simulink model "ejercicio51listo"  (R2017a)
settings: Solver=FixedStepAuto  StartTime=0.0  StopTime=3  FixedStep=1e-6  RelTol=1e-3
undefined symbols (not defined in the file): filtrovco
libraries: dsparch4 x2, commsynccomp2 x1
settings Model: Creator=Nahuel  LastModifiedBy=gusta

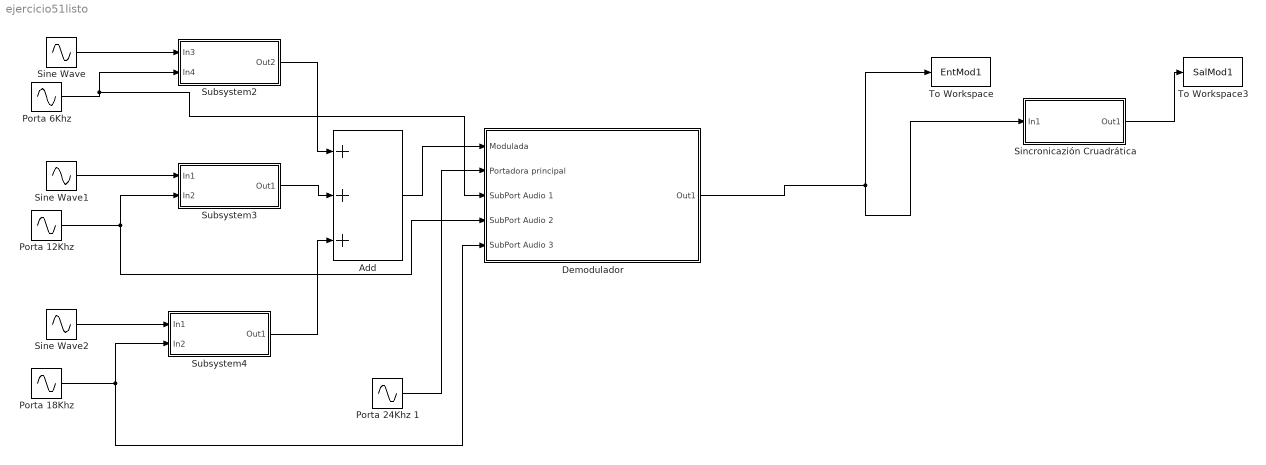
== system ejercicio51listo ==
  Add : Sum  Inputs=+++
  Demodulador : Subsystem
  "Porta 12Khz " : Sin  Frequency=2*pi*12000
  "Porta 18Khz " : Sin  Frequency=2*pi*18000
  Porta 24Khz 1 : Sin  Frequency=2*pi*24000
  "Porta 6Khz " : Sin  Frequency=2*pi*6000
  Sincronicazión Cruadrática : Subsystem
  Sine Wave : Sin  Frequency=100*pi*2  Phase=pi/2
  Sine Wave1 : Sin  Frequency=500*pi*2  Phase=pi/2
  Sine Wave2 : Sin  Frequency=250*pi*2  Phase=pi/2
  Subsystem2 : Subsystem
  Subsystem3 : Subsystem
  Subsystem4 : Subsystem
  To Workspace : ToWorkspace  VariableName=EntMod1  SampleTime=-1
  To Workspace3 : ToWorkspace  VariableName=SalMod1  SampleTime=-1
  wires:
  Demodulador/1(Out1) -> Sincronicazión Cruadrática/1(In1), To Workspace/1
  Sincronicazión Cruadrática/1(Out1) -> To Workspace3/1
  "Porta 6Khz "/1 -> Demodulador/3(SubPort Audio 1), Subsystem2/2(In4)
  Sine Wave/1 -> Subsystem2/1(In3)
  Subsystem2/1(Out2) -> Add/1
  Subsystem3/1(Out1) -> Add/2
  "Porta 12Khz "/1 -> Subsystem3/2(In2), Demodulador/4(SubPort Audio 2)
  Sine Wave1/1 -> Subsystem3/1(In1)
  Subsystem4/1(Out1) -> Add/3
  Sine Wave2/1 -> Subsystem4/1(In1)
  "Porta 18Khz "/1 -> Demodulador/5(SubPort Audio 3), Subsystem4/2(In2)
  Porta 24Khz 1/1 -> Demodulador/2(Portadora principal)
  Add/1 -> Demodulador/1(Modulada)

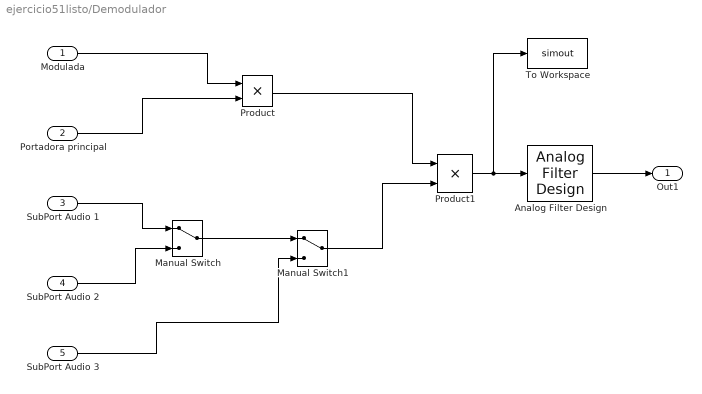
== system ejercicio51listo/Demodulador ==
  Modulada : Inport
  Portadora principal : Inport  Port=2
  SubPort Audio 1 : Inport  Port=3
  SubPort Audio 2 : Inport  Port=4
  SubPort Audio 3 : Inport  Port=5
  Analog Filter Design : dsparch4/Analog Filter Design  method=Butterworth  filttype=Lowpass  N=12  Wlo=2*pi*5000  Whi=80  Rp=2  Rs=40
  Manual Switch : ManualSwitch
  Manual Switch1 : ManualSwitch
  Product : Product
  Product1 : Product
  To Workspace : ToWorkspace  VariableName=simout  SampleTime=-1
  Out1 : Outport
  wires:
  Modulada/1 -> Product/1
  Portadora principal/1 -> Product/2
  Product/1 -> Product1/1
  SubPort Audio 1/1 -> Manual Switch/1
  SubPort Audio 2/1 -> Manual Switch/2
  SubPort Audio 3/1 -> Manual Switch1/2
  Manual Switch1/1 -> Product1/2
  Manual Switch/1 -> Manual Switch1/1
  Product1/1 -> To Workspace/1, Analog Filter Design/1
  Analog Filter Design/1 -> Out1/1

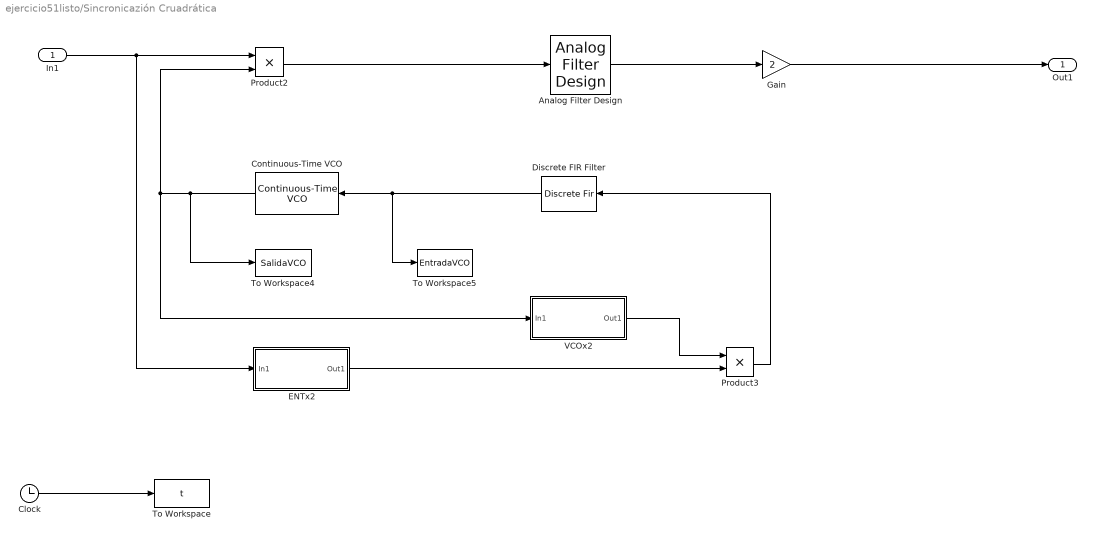
== system ejercicio51listo/Sincronicazión Cruadrática ==
  In1 : Inport
  Analog Filter Design : dsparch4/Analog Filter Design  method=Butterworth  filttype=Lowpass  N=8  Wlo=2*pi*5000  Whi=80  Rp=2  Rs=40
  Clock : Clock
  Continuous-Time VCO : commsynccomp2/Continuous-Time VCO  Ac=1  Fc=fvco  Kc=75  Ph=0
      settings: SourceProductName=Communications System Toolbox  SourceProductBaseCode=CM
  Discrete FIR Filter : DiscreteFir  Coefficients=filtrovco
  ENTx2 : Subsystem
  Gain : Gain  Gain=2
  Product2 : Product
  Product3 : Product
  To Workspace : ToWorkspace  VariableName=t  SampleTime=-1
  To Workspace4 : ToWorkspace  VariableName=SalidaVCO  SampleTime=-1
  To Workspace5 : ToWorkspace  VariableName=EntradaVCO  SampleTime=-1
  VCOx2 : Subsystem
  Out1 : Outport
  wires:
  Discrete FIR Filter/1 -> To Workspace5/1, Continuous-Time VCO/1
  Product2/1 -> Analog Filter Design/1
  Continuous-Time VCO/1 -> To Workspace4/1, VCOx2/1(In1), Product2/2
  Gain/1 -> Out1/1
  Product3/1 -> Discrete FIR Filter/1
  ENTx2/1(Out1) -> Product3/2
  VCOx2/1(Out1) -> Product3/1
  Analog Filter Design/1 -> Gain/1
  In1/1 -> Product2/1, ENTx2/1(In1)
  Clock/1 -> To Workspace/1

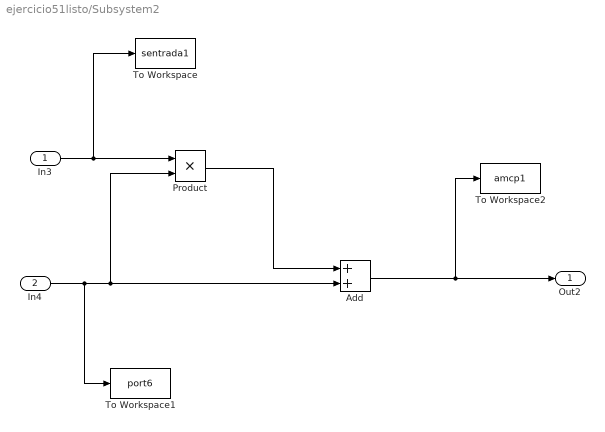
== system ejercicio51listo/Subsystem2 ==
  In3 : Inport
  In4 : Inport  Port=2
  Add : Sum
  Product : Product
  To Workspace : ToWorkspace  VariableName=sentrada1  SampleTime=-1
  To Workspace1 : ToWorkspace  VariableName=port6  SampleTime=-1
  To Workspace2 : ToWorkspace  VariableName=amcp1  SampleTime=-1
  Out2 : Outport
  wires:
  Product/1 -> Add/1
  In3/1 -> To Workspace/1, Product/1
  In4/1 -> To Workspace1/1, Product/2, Add/2
  Add/1 -> To Workspace2/1, Out2/1

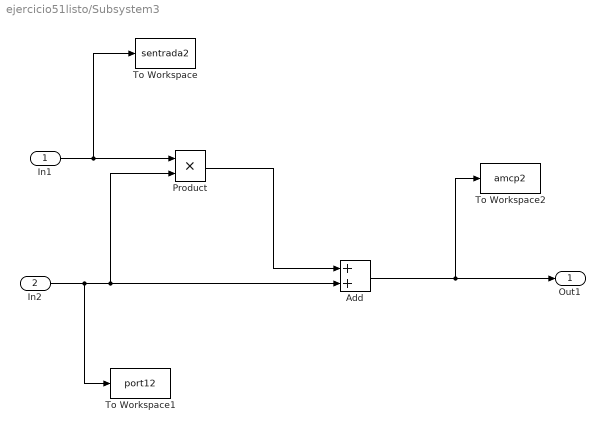
== system ejercicio51listo/Subsystem3 ==
  In1 : Inport
  In2 : Inport  Port=2
  Add : Sum
  Product : Product
  To Workspace : ToWorkspace  VariableName=sentrada2  SampleTime=-1
  To Workspace1 : ToWorkspace  VariableName=port12  SampleTime=-1
  To Workspace2 : ToWorkspace  VariableName=amcp2  SampleTime=-1
  Out1 : Outport
  wires:
  Product/1 -> Add/1
  In1/1 -> To Workspace/1, Product/1
  In2/1 -> To Workspace1/1, Product/2, Add/2
  Add/1 -> To Workspace2/1, Out1/1

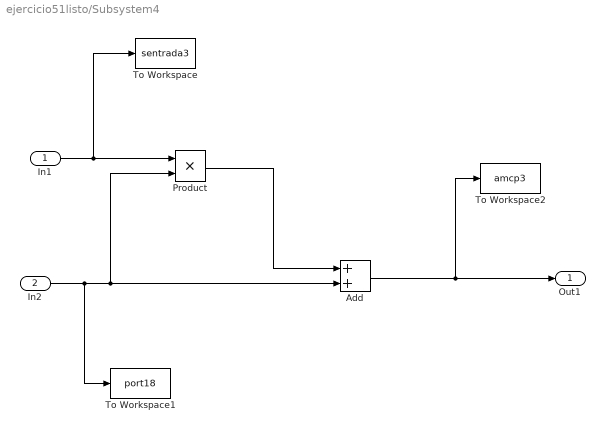
== system ejercicio51listo/Subsystem4 ==
  In1 : Inport
  In2 : Inport  Port=2
  Add : Sum
  Product : Product
  To Workspace : ToWorkspace  VariableName=sentrada3  SampleTime=-1
  To Workspace1 : ToWorkspace  VariableName=port18  SampleTime=-1
  To Workspace2 : ToWorkspace  VariableName=amcp3  SampleTime=-1
  Out1 : Outport
  wires:
  Product/1 -> Add/1
  In1/1 -> To Workspace/1, Product/1
  In2/1 -> To Workspace1/1, Product/2, Add/2
  Add/1 -> To Workspace2/1, Out1/1

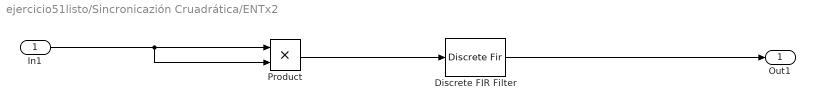
== system ejercicio51listo/Sincronicazión Cruadrática/ENTx2 ==
  In1 : Inport
  Discrete FIR Filter : DiscreteFir
  Product : Product
  Out1 : Outport
  wires:
  In1/1 -> Product/2, Product/1
  Product/1 -> Discrete FIR Filter/1
  Discrete FIR Filter/1 -> Out1/1

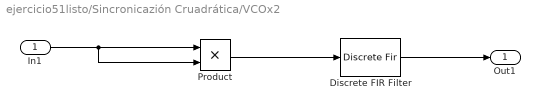
== system ejercicio51listo/Sincronicazión Cruadrática/VCOx2 ==
  In1 : Inport
  Discrete FIR Filter : DiscreteFir
  Product : Product
  Out1 : Outport
  wires:
  In1/1 -> Product/2, Product/1
  Discrete FIR Filter/1 -> Out1/1
  Product/1 -> Discrete FIR Filter/1
